simulink model "FINAL_MODEL"  (R2018a)
settings: Solver=FixedStepAuto  StartTime=startTime  StopTime=stopTime  FixedStep=stepSize  RelTol=1e-3
values from neighbouring files (symbols this model uses):
  burnCount = 2    [AA279D_FINAL.m]
  D2R = pi/180    (= 0.0174532925199)    [AA279D_FINAL.m]    (also in AA279D_PSET2.m; AA279D_PSET2_a_change.m; AA279D_PSET3.m; AA279D_PSET4.m)
  dV = zeros(3)    [AA279D_FINAL.m]    (also in AA279D_PSET2.m = [0;0;0]; AA279D_PSET2_a_change.m = [DVx;DVy;DVz]/stepSize; AA279D_PSET4.m = [0;0;0]; AA279D_hw4_v2.m = [0;0;0])
  dV_Timer = 5    [AA279D_FINAL.m]
  J2 = 1.081874*10^-3    (= 0.001081874)    [AA279D_FINAL.m]    (also in AA279D_PSET1.m; AA279D_PSET2.m; AA279D_PSET2_a_change.m; AA279D_PSET3.m)
  mu = 398600    [AA279D_FINAL.m]    (also in AA279D_PSET1.m; AA279D_PSET2.m; AA279D_PSET2_a_change.m; AA279D_PSET3.m)
  n = n_D    [AA279D_hw4.m]    (also in AA279D_hw4_v2.m = sqrt(mu/a^3); AA279D_hw5_dv.m = sqrt(mu/at^3); OE2ECI.m = sqrt(mu/a^3); TLE_Reader.m = revs_per_day*2*pi/(24*3600))
  Q_LQR = 1/(10)^2*eye(6)    [AA279D_FINAL.m]
  R_LQR = 1/(0.1)^2*eye(3)    [AA279D_FINAL.m]
  Re = 6378137*10^-3    (= 6378.137)    [AA279D_FINAL.m]    (also in AA279D_PSET1.m; AA279D_PSET2.m; AA279D_PSET2_a_change.m; AA279D_PSET3.m)
  roe = roe_out(end,:)    [AA279D_FINAL.m]    (also in AA279D_hw5.m = [0,100,50,100,30,200]/a*10e-4; AA279D_hw5_dv.m = [0,100,50,100,0,200]/a*10e-4; oe2roe.m = [da; deg2rad(dl); deg2rad(dex); deg2rad(dey); deg2rad(dix); )
  sig0 = sig_out(:,:,end)    [AA279D_FINAL.m]
  startTime = stopTime+stepSize    (= 12505)    [AA279D_FINAL.m]
  stepSize = 5    [AA279D_FINAL.m]    (also in AA279D_PSET1.m = 1; AA279D_PSET2.m; AA279D_PSET2_a_change.m = 1; AA279D_PSET3.m)
  uM = mod(uM,2*pi)    [AA279D_FINAL.m]
undefined symbols (not defined in the file or in its folder): r_eci_C, r_eci_D, v_eci_C, v_eci_D
libraries: simulink x3
settings Model: PacingRate=40  Creator=Christopher Covert  LastModifiedBy=Christopher Covert
settings SolverCC: AlgebraicLoopSolver=LineSearch

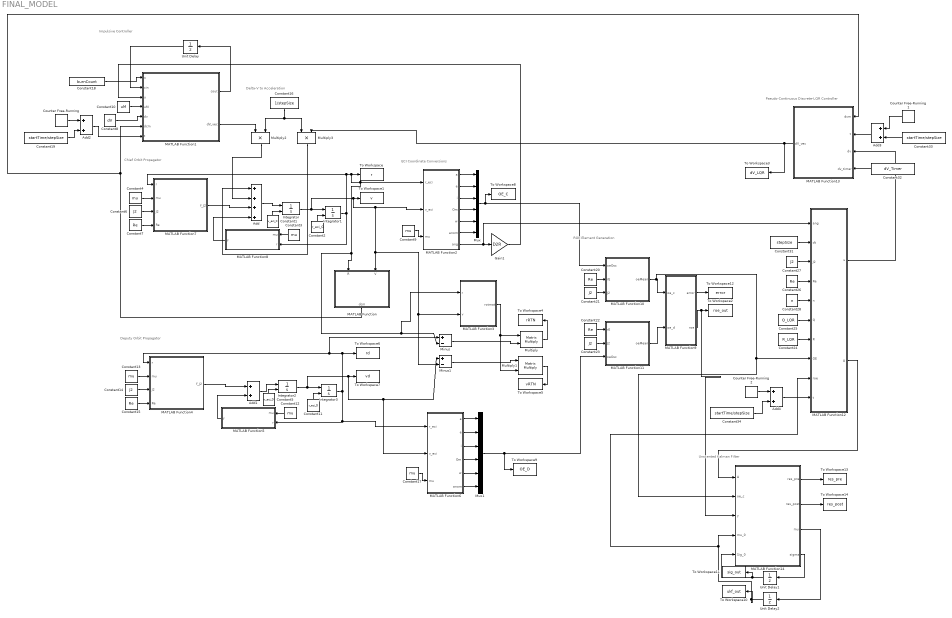
== system FINAL_MODEL ==
  note: Delta-V to Acceleration
  note: Unscented Kalman Filter
  note: Impulsive Controller
  note: Pseudo-Continuous Discrete-LQR Controller
  note: ROE Element Generation
  note: ECI Coordinate Conversions
  note: Chief Orbit Propagator
  note: Deputy Orbit Propagator
  Add : Sum  Inputs=++++
  Add{1..4} (4 alike) : Sum
  Constant1 : Constant  Value=v_eci_C
  Constant10 : Constant  Value=uM
  Constant11 : Constant  Value=r_eci_D
  Constant{3..4,9,12..13,17} (6 alike) : Constant  Value=mu
  Constant{6,14,21,23,27} (5 alike) : Constant  Value=J2
  Constant{7,15,20,22,26} (5 alike) : Constant  Value=Re
  Constant16 : Constant  Value=1/stepSize
  Constant18 : Constant  Value=burnCount
  Constant19 : Constant  Value=startTime/stepSize
  Constant2 : Constant  Value=r_eci_C
  Constant24 : Constant  Value=R_LQR
  Constant25 : Constant  Value=Q_LQR
  Constant28 : Constant  Value=n
  Constant31 : Constant  Value=stepSize
  Constant32 : Constant  Value=dV_Timer
  Constant33 : Constant  Value=startTime/stepSize
  Constant34 : Constant  Value=startTime/stepSize
  Constant5 : Constant  Value=v_eci_D
  Constant8 : Constant  Value=dV
  Counter Free-Running : simulink/Sources/Counter Free-Running  NumBits=16  tsamp=stepSize
  Counter Free-Running1 : simulink/Sources/Counter Free-Running  NumBits=16  tsamp=stepSize
  Counter Free-Running2 : simulink/Sources/Counter Free-Running  NumBits=16  tsamp=stepSize
  Gain1 : Gain  Gain=D2R
  Integrator{,1..3} (4 alike) : Integrator  InitialConditionSource=external
  MATLAB Function : MATLAB Function  TreatAsAtomicUnit=on
  MATLAB Function1 : MATLAB Function  TreatAsAtomicUnit=on
  MATLAB Function10 : MATLAB Function  TreatAsAtomicUnit=on
  MATLAB Function11 : MATLAB Function  TreatAsAtomicUnit=on
  MATLAB Function12 : MATLAB Function  TreatAsAtomicUnit=on
  MATLAB Function13 : MATLAB Function  TreatAsAtomicUnit=on
  MATLAB Function14 : MATLAB Function  TreatAsAtomicUnit=on
  MATLAB Function2 : MATLAB Function  TreatAsAtomicUnit=on
  MATLAB Function3 : MATLAB Function  TreatAsAtomicUnit=on
  MATLAB Function4 : MATLAB Function  TreatAsAtomicUnit=on
  MATLAB Function5 : MATLAB Function  TreatAsAtomicUnit=on
  MATLAB Function6 : MATLAB Function  TreatAsAtomicUnit=on
  MATLAB Function7 : MATLAB Function  TreatAsAtomicUnit=on
  MATLAB Function8 : MATLAB Function  TreatAsAtomicUnit=on
  MATLAB Function9 : MATLAB Function  TreatAsAtomicUnit=on
  Minus : Sum  Inputs=+-
  Minus1 : Sum  Inputs=+-
  Multiply : Product  Multiplication=Matrix(*)
  Multiply1 : Product  Multiplication=Matrix(*)
  Multiply2 : Product
  Multiply3 : Product
  Mux : Mux  Inputs=6
  Mux1 : Mux  Inputs=6
  To Workspace : ToWorkspace  VariableName=r  SampleTime=-1
      settings: Save2DSignal=2-D array (concatenate along first dimension)
  To Workspace1 : ToWorkspace  VariableName=v  SampleTime=-1
      settings: Save2DSignal=2-D array (concatenate along first dimension)
  To Workspace10 : ToWorkspace  VariableName=ukf_out  SampleTime=-1
      settings: Save2DSignal=2-D array (concatenate along first dimension)
  To Workspace11 : ToWorkspace  VariableName=sig_out  SampleTime=-1
  To Workspace12 : ToWorkspace  VariableName=error  SampleTime=-1
      settings: Save2DSignal=2-D array (concatenate along first dimension)
  To Workspace13 : ToWorkspace  VariableName=res_pre  SampleTime=-1
      settings: Save2DSignal=2-D array (concatenate along first dimension)
  To Workspace14 : ToWorkspace  VariableName=res_post  SampleTime=-1
      settings: Save2DSignal=2-D array (concatenate along first dimension)
  To Workspace2 : ToWorkspace  VariableName=roe_out  SampleTime=-1
      settings: Save2DSignal=2-D array (concatenate along first dimension)
  To Workspace3 : ToWorkspace  VariableName=dV_LQR  SampleTime=-1
      settings: Save2DSignal=2-D array (concatenate along first dimension)
  To Workspace4 : ToWorkspace  VariableName=rRTN  SampleTime=-1
      settings: Save2DSignal=2-D array (concatenate along first dimension)
  To Workspace5 : ToWorkspace  VariableName=vRTN  SampleTime=-1
      settings: Save2DSignal=2-D array (concatenate along first dimension)
  To Workspace6 : ToWorkspace  VariableName=rd  SampleTime=-1
      settings: Save2DSignal=2-D array (concatenate along first dimension)
  To Workspace7 : ToWorkspace  VariableName=vd  SampleTime=-1
      settings: Save2DSignal=2-D array (concatenate along first dimension)
  To Workspace8 : ToWorkspace  VariableName=OE_C  SampleTime=-1
      settings: Save2DSignal=2-D array (concatenate along first dimension)
  To Workspace9 : ToWorkspace  VariableName=OE_D  SampleTime=-1
      settings: Save2DSignal=2-D array (concatenate along first dimension)
  Unit Delay : UnitDelay  InputProcessing=Columns as channels (frame based)  SampleTime=-1
  Unit Delay1 : UnitDelay  InitialCondition=sig0  SampleTime=stepSize
  Unit Delay2 : UnitDelay  InitialCondition=roe  SampleTime=stepSize
  wires:
  Integrator/1 -> Integrator1/1, Minus1/2, MATLAB Function3/2(v), MATLAB Function/2(V), MATLAB Function2/2(v_eci), To Workspace1/1
  Constant3/1 -> MATLAB Function8/1(mu)
  Constant4/1 -> MATLAB Function7/2(mu)
  Constant6/1 -> MATLAB Function7/3(J2)
  Add/1 -> Integrator/1
  Constant7/1 -> MATLAB Function7/4(Re)
  MATLAB Function8/1(f) -> Add/4
  MATLAB Function7/1(f_J2) -> Add/3
  Constant1/1 -> Integrator/2
  Constant2/1 -> Integrator1/2
  Multiply2/1 -> Add/2
  MATLAB Function2/7(ang) -> MATLAB Function12/1(ang), Gain1/1
  Constant8/1 -> MATLAB Function1/5(dv)
  MATLAB Function1/2(dV_vec) -> Multiply2/1
  Constant9/1 -> MATLAB Function2/3(mu)
  Unit Delay/1 -> MATLAB Function1/2(cin)
  MATLAB Function1/1(cout) -> Unit Delay/1
  Constant10/1 -> MATLAB Function1/4(uM)
  MATLAB Function/1(dcm) -> MATLAB Function13/1(dcm), MATLAB Function1/6(dcm)
  MATLAB Function2/1(a) -> Mux/1
  MATLAB Function2/2(e) -> Mux/2
  MATLAB Function2/3(i) -> Mux/3
  MATLAB Function2/4(Om) -> Mux/4
  MATLAB Function2/5(w) -> Mux/5
  MATLAB Function2/6(anom) -> Mux/6
  Mux/1 -> To Workspace8/1, MATLAB Function10/1(oeOsc)
  Gain1/1 -> MATLAB Function1/3(u)
  Multiply1/1 -> To Workspace5/1
  Constant13/1 -> MATLAB Function4/2(mu)
  Constant15/1 -> MATLAB Function4/4(Re)
  Constant12/1 -> MATLAB Function5/1(mu)
  Constant5/1 -> Integrator2/2
  Constant11/1 -> Integrator3/2
  Constant14/1 -> MATLAB Function4/3(J2)
  Add1/1 -> Integrator2/1
  MATLAB Function4/1(f_J2) -> Add1/1
  MATLAB Function5/1(f) -> Add1/2
  Minus/1 -> Multiply/2
  Minus1/1 -> Multiply1/1
  Integrator1/1 -> MATLAB Function8/2(r), MATLAB Function7/1(r), MATLAB Function3/1(r), Minus/2, MATLAB Function/1(R), MATLAB Function2/1(r_eci), To Workspace/1
  MATLAB Function3/1(rotmat) -> Multiply1/2, Multiply/1
  Multiply/1 -> To Workspace4/1
  Constant16/1 -> Multiply2/2, Multiply3/1
  MATLAB Function6/6(anom) -> Mux1/6
  Integrator2/1 -> Integrator3/1, MATLAB Function6/2(v_eci), Minus1/1, To Workspace7/1
  Integrator3/1 -> MATLAB Function6/1(r_eci), MATLAB Function5/2(r), Minus/1, MATLAB Function4/1(r), To Workspace6/1
  Constant17/1 -> MATLAB Function6/3(mu)
  MATLAB Function6/3(i) -> Mux1/3
  MATLAB Function6/5(w) -> Mux1/5
  MATLAB Function6/1(a) -> Mux1/1
  MATLAB Function6/2(e) -> Mux1/2
  MATLAB Function6/4(Om) -> Mux1/4
  Counter Free-Running/1 -> Add2/1
  Constant19/1 -> Add2/2
  Add2/1 -> MATLAB Function1/7(t)
  Constant18/1 -> MATLAB Function1/1(n)
  MATLAB Function10/1(oeMean) -> MATLAB Function14/2(oe_c), MATLAB Function12/8(OE), MATLAB Function9/1(oe_c)
  Constant20/1 -> MATLAB Function10/2(rE)
  Constant21/1 -> MATLAB Function10/3(J2)
  Constant22/1 -> MATLAB Function11/1(rE)
  Constant23/1 -> MATLAB Function11/2(J2)
  Mux1/1 -> MATLAB Function11/3(oeOsc), To Workspace9/1
  MATLAB Function11/1(oeMean) -> MATLAB Function9/2(oe_d)
  MATLAB Function9/2(roe) -> MATLAB Function14/3(y), To Workspace2/1
  Constant24/1 -> MATLAB Function12/7(R)
  Constant25/1 -> MATLAB Function12/6(Q)
  Constant26/1 -> MATLAB Function12/4(Re)
  Constant27/1 -> MATLAB Function12/3(J2)
  MATLAB Function12/1(u) -> MATLAB Function13/3(dv)
  Constant28/1 -> MATLAB Function12/5(n)
  MATLAB Function13/1(dV_vec) -> To Workspace3/1, Multiply3/2
  Multiply3/1 -> Add/1
  Constant31/1 -> MATLAB Function12/2(dt)
  Constant33/1 -> Add3/2
  Counter Free-Running1/1 -> Add3/1
  Constant32/1 -> MATLAB Function13/4(dv_timer)
  Add3/1 -> MATLAB Function13/2(t)
  Constant34/1 -> Add4/2
  Counter Free-Running2/1 -> Add4/1
  Add4/1 -> MATLAB Function12/10(t)
  MATLAB Function14/4(sigma) -> Unit Delay1/1
  MATLAB Function14/3(mu) -> Unit Delay2/1
  Unit Delay1/1 -> MATLAB Function14/5(Sig_0), To Workspace11/1
  MATLAB Function12/2(A) -> MATLAB Function14/1(A)
  MATLAB Function14/1(res_pre) -> To Workspace13/1
  MATLAB Function14/2(res_post) -> To Workspace14/1
  Unit Delay2/1 -> To Workspace10/1, MATLAB Function12/9(roe), MATLAB Function14/4(mu_0)
  MATLAB Function9/1(error) -> To Workspace12/1

== matlab function FINAL_MODEL/MATLAB Function1 ==
  data: n input; cin input; u input; uM input; cout output; dv input; dV_vec output; dcm input; t input
function [cout,dV_vec] = impulse_man(n,cin,u,uM,dv,dcm,t)

i = cin+1;

if double(t) == 116 && n == 1
    dV_vec = dcm*[dv(1,1);dv(2,1);dv(3,1)];
%     fprintf('Completed Burn No.%0.0f at t = %0.2f\n',i,double(t));
    cout = cin+1;
elseif n == 2 && double(t) == 3519
    dV_vec = dcm*[dv(1,1);dv(2,1);dv(3,1)];
%     fprintf('Completed Burn No.%0.0f at t = %0.2f\n',i,double(t));
    cout = cin+1;
elseif double(t) == 830 && n == 1
    dV_vec = -dcm*[dv(1,2);dv(2,2);dv(3,2)];
%     fprintf('Completed Burn No.%0.0f at t = %0.2f\n',i,double(t));
    cout = cin+1;
elseif  n == 2 && double(t) == 4130
    dV_vec = -dcm*[dv(1,2);dv(2,2);dv(3,2)]*1.1;
%     fprintf('Completed Burn No.%0.0f at t = %0.2f\n',i,double(t));
    cout = cin+1;
elseif double(t) == 1385 && n == 1
    dV_vec = -dcm*[dv(1,3);dv(2,3);dv(3,3)];
%     fprintf('Completed Burn No.%0.0f at t = %0.2f\n',i,double(t));
    cout = cin+1;
elseif  n == 2 && double(t) == 4673
    dV_vec = -dcm*[dv(1,3);dv(2,3);dv(3,3)]*0.93;
%     fprintf('Completed Burn No.%0.0f at t = %0.2f\n',i,double(t));
    cout = cin+1;
else
    dV_vec = [0;0;0];
    cout = cin;
end

end

== matlab function FINAL_MODEL/MATLAB Function2 ==
  data: a output; e output; i output; Om output; r_eci input; v_eci input; mu input; w output; anom output; ang output
function [a, e, i, Om, w, anom, ang] = ECI2OE(r_eci, v_eci, mu)
% ECI2OE Converts r and v in the ECI frame to orbital elements
%
% Inputs:
%   r_eci - 3x1 vector of radius in ECI frame [km]
%   v_eci - 3x1 vector of velocity in ECI frame [km]
%   mu    - gravitational parameter of central body [km^3/s^2]
%
% Outputs:
%   p     - semi-lactus rectum of orbit [km]
%   a     - semi-major axis of orbit [km]
%   e     - eccentricity of orbit
%   i     - inclination of orbit [deg]
%   Om    - right ascension of the ascending node [deg]
%   w     - argument of periapsis [deg]
%   v     - true anomaly [deg]
%   ang   - extra placeholder angle for special cases [deg]
%
% This function is able to handle any orbit type, including equatorial and
% circular orbits. The output ang will output the following values for each
% orbit type
%   1) Elliptical equatorial
%       Longitude of periapsis, Pi = Om + w
%   2) Circular inclined
%       Argument of latitude, u = w + anom
%   3) Circular equatorial
%       True latitude, lambda = Om + w + anom
% Otherwise, ang will be undefined (NaN)

r = norm(r_eci);
v = norm(v_eci);

% Create all necessary vectors
hVec = cross(r_eci, v_eci);
h = norm(hVec);

nVec = cross([0, 0, 1], hVec);
n = norm(nVec);

eVec = (1/mu)*((v^2 - mu/r)*r_eci - dot(r_eci, v_eci)*v_eci);
e = norm(eVec);

% Compute the size of the orbit
mechEnergy = 0.5*v^2 - mu/r;

if e ~= 1
    a = -mu/(2*mechEnergy);
else
    a = inf; % Semi-major axis undefined for parabolas
end

% Compute the orientation of the orbit
i = rad2deg(acos(hVec(3)/h));
Om = rad2deg(acos(nVec(1)/n));
w = rad2deg(acos(dot(nVec, eVec)/(n*e)));
anom = rad2deg(acos(dot(eVec, r_eci)/(e*r)));

% Place angles in the correct domains
if nVec(2) < 0
    Om = 360 - Om;
end
if eVec(3) < 0
    w = 360 - w;
end
if dot(r_eci, v_eci) < 0
    anom = 360 - anom;
end

% Account for any special cases
if i == 0 && e ~= 0 % Elliptical equatorial
    % Provide the longitude of periapsis (PI = Om + w)
    ang = rad2deg(acos(eVec(1)/e));

    if eVec(2) < 0
        ang = 360 - ang;
    end
elseif i ~= 0 && e == 0 % Circular inclined
    % Provide the argument of latitude (u = w + anom)
    ang = rad2deg(acos(dot(nVec, r_eci)/(n*r)));

    if r_eci(3) < 0
        ang = 360 - ang;
    end
elseif i == 0 && e == 0 % Circular equatorial
    % Provide the true latitude (lambda = Om + w + anom)
    ang = rad2deg(acos(r_eci(1)/r));

    if r_eci(2) < 0
        ang = 360 - ang;
    end
else
    % Default output for ang
    ang = NaN;
end

ang = mod(w + anom,360);


end

== matlab function FINAL_MODEL/MATLAB Function ==
  data: R input; dcm output; V input
function dcm = RTN2ECI(R, V)
% RTN2ECI Computes rotation matrices from RTN frame to inertial frame
%
% Inputs:
%   R - 3xn inertial position vectors
%   V - 3xn inertial velocity vectors
%
% Outputs:
%   dcm - 3x3xn rotation matrices from inertial to RTN

% Set up the input matrices as a (3 x n) series of column vectors
if size(R, 2) == 3 && size(R, 1) ~= 3
    R = R.';
end

if size(V, 2) == 3 && size(V, 1) ~= 3
    V = V.';
end

% Check input sizes
numPos = size(R, 2);
numVel = size(V, 2);

if size(R, 1) ~= 3
    error('Position vectors must come in the form of 3xn column vectors');
elseif size(V, 1) ~= 3
    error('Velocity vectors must come in the form of 3xn column vectors');
elseif numPos ~= numVel
    error('Must provide the same number of position and velocity vectors');
end

dcm = zeros(3, 3, numPos);

for i = 1:numPos
    rVec = R(:, i)./norm(R(:, i));
    
    H = cross(R(:, i), V(:, i));
    nVec = H./norm(H);
    
    T = cross(nVec, rVec);
    tVec = T./norm(T);
    
    dcm(:, :, i) = [rVec, tVec, nVec];
end

end

== matlab function FINAL_MODEL/MATLAB Function7 ==
  data: r input; f_J2 output; mu input; J2 input; Re input
function f_J2 = J2_Accel(r,mu,J2,Re)

f_J2 = mu*r/(norm(r)^3).*...
    [3/2*J2*(Re/norm(r))^2*(5*(r(3)^2)/(norm(r)^2)-1);...
    3/2*J2*(Re/norm(r))^2*(5*(r(3)^2)/(norm(r)^2)-1);...
    3/2*J2*(Re/norm(r))^2*(5*(r(3)^2)/(norm(r)^2)-3)];

== matlab function FINAL_MODEL/MATLAB Function8 ==
  data: mu input; f output; r input
function f = FODE_NUM_PROP(mu,r)

f = -mu*r/(norm(r)^3);

== matlab function FINAL_MODEL/MATLAB Function3 ==
  data: r input; rotmat output; v input
function rotmat = ECI2RTN( r,v)

r=reshape(r,1,3);
v=reshape(v,1,3);
unitr=r/norm(r);
unitn=cross(r,v)/norm(cross(r,v));
unitt=cross(unitn,r)/norm(cross(unitn,r));
rotmat=[unitr;
    unitt;
    unitn];

end

== matlab function FINAL_MODEL/MATLAB Function4 ==
  data: r input; f_J2 output; mu input; J2 input; Re input
function f_J2 = J2_Accel(r,mu,J2,Re)

f_J2 = mu*r/(norm(r)^3).*...
    [3/2*J2*(Re/norm(r))^2*(5*(r(3)^2)/(norm(r)^2)-1);...
    3/2*J2*(Re/norm(r))^2*(5*(r(3)^2)/(norm(r)^2)-1);...
    3/2*J2*(Re/norm(r))^2*(5*(r(3)^2)/(norm(r)^2)-3)];

== matlab function FINAL_MODEL/MATLAB Function5 ==
  data: mu input; f output; r input
function f = FODE_NUM_PROP(mu,r)

f = -mu*r/(norm(r)^3);

== matlab function FINAL_MODEL/MATLAB Function6 ==
  data: a output; e output; i output; Om output; r_eci input; v_eci input; mu input; w output; anom output
function [a, e, i, Om, w, anom] = ECI2OE(r_eci, v_eci, mu)
% ECI2OE Converts r and v in the ECI frame to orbital elements
%
% Inputs:
%   r_eci - 3x1 vector of radius in ECI frame [km]
%   v_eci - 3x1 vector of velocity in ECI frame [km]
%   mu    - gravitational parameter of central body [km^3/s^2]
%
% Outputs:
%   p     - semi-lactus rectum of orbit [km]
%   a     - semi-major axis of orbit [km]
%   e     - eccentricity of orbit
%   i     - inclination of orbit [deg]
%   Om    - right ascension of the ascending node [deg]
%   w     - argument of periapsis [deg]
%   v     - true anomaly [deg]
%   ang   - extra placeholder angle for special cases [deg]
%
% This function is able to handle any orbit type, including equatorial and
% circular orbits. The output ang will output the following values for each
% orbit type
%   1) Elliptical equatorial
%       Longitude of periapsis, Pi = Om + w
%   2) Circular inclined
%       Argument of latitude, u = w + anom
%   3) Circular equatorial
%       True latitude, lambda = Om + w + anom
% Otherwise, ang will be undefined (NaN)

r = norm(r_eci);
v = norm(v_eci);

% Create all necessary vectors
hVec = cross(r_eci, v_eci);
h = norm(hVec);

nVec = cross([0, 0, 1], hVec);
n = norm(nVec);

eVec = (1/mu)*((v^2 - mu/r)*r_eci - dot(r_eci, v_eci)*v_eci);
e = norm(eVec);

% Compute the size of the orbit
mechEnergy = 0.5*v^2 - mu/r;

if e ~= 1
    a = -mu/(2*mechEnergy);
else
    a = inf; % Semi-major axis undefined for parabolas
end

% Compute the orientation of the orbit
i = rad2deg(acos(hVec(3)/h));
Om = rad2deg(acos(nVec(1)/n));
w = rad2deg(acos(dot(nVec, eVec)/(n*e)));
anom = rad2deg(acos(dot(eVec, r_eci)/(e*r)));

% Place angles in the correct domains
if nVec(2) < 0
    Om = 360 - Om;
end
if eVec(3) < 0
    w = 360 - w;
end
if dot(r_eci, v_eci) < 0
    anom = 360 - anom;
end

% Account for any special cases
if i == 0 && e ~= 0 % Elliptical equatorial
    % Provide the longitude of periapsis (PI = Om + w)
    ang = rad2deg(acos(eVec(1)/e));

    if eVec(2) < 0
        ang = 360 - ang;
    end
elseif i ~= 0 && e == 0 % Circular inclined
    % Provide the argument of latitude (u = w + anom)
    ang = rad2deg(acos(dot(nVec, r_eci)/(n*r)));

    if r_eci(3) < 0
        ang = 360 - ang;
    end
elseif i == 0 && e == 0 % Circular equatorial
    % Provide the true latitude (lambda = Om + w + anom)
    ang = rad2deg(acos(r_eci(1)/r));

    if r_eci(2) < 0
        ang = 360 - ang;
    end
else
    % Default output for ang
    ang = NaN;
end

ang = mod(w + anom,360);


end

== matlab function FINAL_MODEL/MATLAB Function9 ==
  data: error output; oe_c input; roe output; oe_d input
function [error,roe]  = oe2roe(oe_c, oe_d)
% oe2roe Converts absolute to relative orbital elements
%
% Inputs:
%       oe_c - chief orbital elements (all angles in degrees)
%              [a, e, i, Om, w, anom]
%       oe_d - deputy orbital elements (all angles in degrees)
%              [ad, ed, id, Omd, wd, anomd]
%   anomFlag - (optional) flag indicating whether the provided anomalies
%              are true (1 - default) or mean (0). The output set of deputy
%              OEs will match.
%
% Outputs:
%        roe - quasi-non singular relative orbital elements

% Parse out the chief and deputy orbit elements
a = oe_c(1);
e = oe_c(2);
i = oe_c(3);
Om = oe_c(4);
w = oe_c(5);
anom = oe_c(6);

ad = oe_d(1);
ed = oe_d(2);
id = oe_d(3);
Omd = oe_d(4);
wd = oe_d(5);
anomd = oe_d(6);

M = rad2deg(E2M(anom2E(deg2rad(anom), e), e));
Md = rad2deg(E2M(anom2E(deg2rad(anomd), ed), ed));

u = w + M;
ud = wd + Md;

Om_diff = Omd-Om;

if Om_diff < -340
    Om_diff = Om_diff + 360;
end

% Compute D'Amico's quasi-nonsingular ROEs
da = (ad - a)./a;
dl = (ud - u) + (Om_diff).*cosd(i);
dex = ed.*cosd(wd) - e.*cosd(w);
dey = ed.*sind(wd) - e.*sind(w);
dix = id - i;
diy = (Om_diff).*sind(i);

error = Omd-Om;

if dl > 340
    dl = dl-360;
end

if dl < -340
    dl = dl+360;
end

roe = [da; deg2rad(dl); deg2rad(dex); deg2rad(dey); deg2rad(dix); deg2rad(diy)];

end

== matlab function FINAL_MODEL/MATLAB Function10 ==
  data: oeOsc input; oeMean output; rE input; J2 input
function oeMean = osc2mean(oeOsc, rE, J2)
% osc2mean Converts osculating orbit elements to mean orbit elements
%
%   This method is based on the first-order mapping provided in Schaub
%   Appendix G. Note that it only accounts for first-order J2 terms, and
%   thus cannot be applied to any general set of osculating orbit elements.
%
%   Note that this method fails for perfectly circular/equatorial orbits.
%   It is recommended that a very small offset (e.g. 1E-6) is introduced to
%   the eccentricity/inclination if one wishes to evaluate the conversion
%   for a circular/equatorial orbit.
%
% Inputs:
%   oeOsc - 6x1 vector of osculating orbit elements:
%          a - semi-major axis of osculating orbit [km]
%          e - eccentricity of osculating orbit
%          i - inclination of osculating orbit [deg]
%         Om - osculating right ascension of the ascending node [deg]
%          w - osculating argument of periapsis [deg]
%       anom - osculating true anomaly [deg]
%     rE - equatorial radius of central body [km]
%     J2 - central body J2 term
%
% Outputs:
%   oeMean - 6x1 vector of mean orbit elements:
%          a - semi-major axis of mean orbit [km]
%          e - eccentricity of mean orbit
%          i - inclination of mean orbit [deg]
%         Om - mean right ascension of the ascending node [deg]
%          w - mean argument of periapsis [deg]
%       anom - mean true anomaly [deg]

% Parse out the osculating orbit elements
a = oeOsc(1);
e = oeOsc(2);
i = oeOsc(3);
Om = oeOsc(4);
w = oeOsc(5);
anom = oeOsc(6);

% Convert all input elements from degrees to radian
i = deg2rad(i);
Om = deg2rad(Om);
w = deg2rad(w);
anom = deg2rad(anom);

% Wrap angles between -pi and pi (robustness)
i = mod(i, pi);
Om = mod(Om, 2*pi) - (Om > pi)*2*pi;
w = mod(w, 2*pi) - (w > pi)*2*pi;
%anom = mod(anom, 2*pi) - (anom > pi)*2*pi;

% Convert the true anomaly to mean anomaly
E = anom2E(anom, e);
M = E2M(E, e);

% Gather necessary constants
g2 = -(J2/2)*(rE/a)^2; % Note: minus sign indicates osc -> mean
eta = sqrt(1 - e^2);
g2_p = g2/eta^4;

a_r = (1 + e*cos(anom))/eta^2;

% Equation G.304:
de1 = (g2_p/8)*e*eta^2*(1 - 11*cos(i)^2 - ...
    40*(cos(i)^4/(1 - 5*cos(i)^2)))*cos(2*w);
de2 = g2*((3*cos(i)^2 - 1)/eta^6)*(e*eta + e/(1 + eta) + ...
    3*cos(anom) + 3*e*cos(anom)^2 + e^2*cos(anom)^3);
de3 = g2*(3*(1 - cos(i)^2)/eta^6)*(e + 3*cos(anom) + ...
    3*e*cos(anom)^2 + e^2*cos(anom)^3)*cos(2*w + 2*anom);
de4 = -g2_p*(1 - cos(i)^2)*(3*cos(2*w + anom) + cos(2*w + 3*anom));

de = de1 + (eta^2)/2*(de2 + de3 + de4);

% Equation G.305:
di1 = -(e*de1)/(eta^2*tan(i));
di2 = g2_p/2*cos(i)*sqrt(1 - cos(i)^2)*(3*cos(2*w + 2*anom) + ...
    3*e*cos(2*w + anom) + e*cos(2*w + 3*anom));

di = di1 + di2;

% Equation G.306:
dL0 = M + w + Om;
dL1 = (g2_p/8)*eta^3*(1 - 11*cos(i)^2 - ...
    40*(cos(i)^4/(1 - 5*cos(i)^2)));
dL2 = -(g2_p/16)*(2 + e^2 - 11*(2 + 3*e^2)*cos(i)^2 - ...
    40*(2 + 5*e^2)*(cos(i)^4/(1 - 5*cos(i)^2)) - ...
    400*e^2*(cos(i)^6/(1 - 5*cos(i)^2)^2));
dL3 = (g2_p/4)*(-6*(1 - 5*cos(i)^2)*(anom - M + e*sin(anom)) + ...
    (3 - 5*cos(i)^2)*(3*sin(2*w + 2*anom) + 3*e*sin(2*w + anom) + ...
    e*sin(2*w + 3*anom)));
dL4 = -(g2_p/8)*e^2*cos(i)*(11 + 80*(cos(i)^2/(1 - 5*cos(i)^2)) +...
    200*(cos(i)^4/(1 - 5*cos(i)^2)^2));
dL5 = -(g2_p/2)*cos(i)*(6*(anom - M + e*sin(anom)) - ...
    3*sin(2*w + 2*anom) - 3*e*sin(2*w + anom) - e*sin(2*w + 3*anom));

dL = dL0 + dL1 + dL2 + dL3 + dL4 + dL5;

% Equation G.307:
edM1 = (g2_p/8)*e*eta^3*(1 - 11*cos(i)^2 - ...
    40*(cos(i)^4/(1 - 5*cos(i)^2)));
edM2 = 2*(3*cos(i)^2 - 1)*((a_r*eta)^2 + a_r + 1)*sin(anom);
edM3 = 3*(1 - cos(i)^2)*((-(a_r*eta)^2 - a_r + 1)*sin(2*w + anom) + ...
    ((a_r*eta)^2 + a_r + 1/3)*sin(2*w + 3*anom));

edM = edM1 - (g2_p/4)*eta^3*(edM2 + edM3);

% Equation G.308
dOm1 = -(g2_p/8)*e^2*cos(i)*(11 + 80*(cos(i)^2/(1 - 5*cos(i)^2)) +...
    200*(cos(i)^4/(1 - 5*cos(i)^2)^2));
dOm2 = -(g2_p/2)*cos(i)*(6*(anom - M + e*sin(anom)) - ...
    3*sin(2*w + 2*anom) - 3*e*sin(2*w + anom) - e*sin(2*w + 3*anom));

dOm = dOm1 + dOm2;

% Equations G.309-310, G.313-314
d1 = (e + de)*sin(M) + edM*cos(M);
d2 = (e + de)*cos(M) - edM*sin(M);
d3 = (sin(i/2) + cos(i/2)*(di/2))*sin(Om) + sin(i/2)*dOm*cos(Om);
d4 = (sin(i/2) + cos(i/2)*(di/2))*cos(Om) - sin(i/2)*dOm*sin(Om);

% Compute all of the mean orbit elements using the previously computed
% parameters
aM = a + a*g2*((3*cos(i)^2 - 1)*(a_r^3 - 1/eta^3) + ...
    3*(1 - cos(i)^2)*a_r^3*cos(2*w + 2*anom));
eM = sqrt(d1^2 + d2^2);
iM = 2*asin(sqrt(d3^2 + d4^2));
OmM = mod(atan2(d3, d4), 2*pi);
MM = mod(atan2(d1, d2), 2*pi);
wM = mod(dL - MM - OmM, 2*pi);

% Convert the mean mean anomaly to mean true anomaly
EM = M2E(MM, e, 1E-9);
anomM = E2anom(EM, e);

% Convert all mean orbit elements from radians to degrees
iM = rad2deg(iM);
OmM = rad2deg(OmM);
wM = rad2deg(wM);
anomM = rad2deg(anomM);

% Gather the mean orbit elements into one vector
oeMean = [aM; eM; iM; OmM; wM; anomM];

end

== matlab function FINAL_MODEL/MATLAB Function11 ==
  data: rE input; J2 input; oeOsc input; oeMean output
function oeMean = osc2mean(  rE, J2, oeOsc)
% osc2mean Converts osculating orbit elements to mean orbit elements
%
%   This method is based on the first-order mapping provided in Schaub
%   Appendix G. Note that it only accounts for first-order J2 terms, and
%   thus cannot be applied to any general set of osculating orbit elements.
%
%   Note that this method fails for perfectly circular/equatorial orbits.
%   It is recommended that a very small offset (e.g. 1E-6) is introduced to
%   the eccentricity/inclination if one wishes to evaluate the conversion
%   for a circular/equatorial orbit.
%
% Inputs:
%   oeOsc - 6x1 vector of osculating orbit elements:
%          a - semi-major axis of osculating orbit [km]
%          e - eccentricity of osculating orbit
%          i - inclination of osculating orbit [deg]
%         Om - osculating right ascension of the ascending node [deg]
%          w - osculating argument of periapsis [deg]
%       anom - osculating true anomaly [deg]
%     rE - equatorial radius of central body [km]
%     J2 - central body J2 term
%
% Outputs:
%   oeMean - 6x1 vector of mean orbit elements:
%          a - semi-major axis of mean orbit [km]
%          e - eccentricity of mean orbit
%          i - inclination of mean orbit [deg]
%         Om - mean right ascension of the ascending node [deg]
%          w - mean argument of periapsis [deg]
%       anom - mean true anomaly [deg]

% Parse out the osculating orbit elements
a = oeOsc(1);
e = oeOsc(2);
i = oeOsc(3);
Om = oeOsc(4);
w = oeOsc(5);
anom = oeOsc(6);

% Convert all input elements from degrees to radian
i = deg2rad(i);
Om = deg2rad(Om);
w = deg2rad(w);
anom = deg2rad(anom);

% Wrap angles between -pi and pi (robustness)
i = mod(i, pi);
Om = mod(Om, 2*pi) - (Om > pi)*2*pi;
w = mod(w, 2*pi) - (w > pi)*2*pi;
%anom = mod(anom, 2*pi) - (anom > pi)*2*pi;

% Convert the true anomaly to mean anomaly
E = anom2E(anom, e);
M = E2M(E, e);

% Gather necessary constants
g2 = -(J2/2)*(rE/a)^2; % Note: minus sign indicates osc -> mean
eta = sqrt(1 - e^2);
g2_p = g2/eta^4;

a_r = (1 + e*cos(anom))/eta^2;

% Equation G.304:
de1 = (g2_p/8)*e*eta^2*(1 - 11*cos(i)^2 - ...
    40*(cos(i)^4/(1 - 5*cos(i)^2)))*cos(2*w);
de2 = g2*((3*cos(i)^2 - 1)/eta^6)*(e*eta + e/(1 + eta) + ...
    3*cos(anom) + 3*e*cos(anom)^2 + e^2*cos(anom)^3);
de3 = g2*(3*(1 - cos(i)^2)/eta^6)*(e + 3*cos(anom) + ...
    3*e*cos(anom)^2 + e^2*cos(anom)^3)*cos(2*w + 2*anom);
de4 = -g2_p*(1 - cos(i)^2)*(3*cos(2*w + anom) + cos(2*w + 3*anom));

de = de1 + (eta^2)/2*(de2 + de3 + de4);

% Equation G.305:
di1 = -(e*de1)/(eta^2*tan(i));
di2 = g2_p/2*cos(i)*sqrt(1 - cos(i)^2)*(3*cos(2*w + 2*anom) + ...
    3*e*cos(2*w + anom) + e*cos(2*w + 3*anom));

di = di1 + di2;

% Equation G.306:
dL0 = M + w + Om;
dL1 = (g2_p/8)*eta^3*(1 - 11*cos(i)^2 - ...
    40*(cos(i)^4/(1 - 5*cos(i)^2)));
dL2 = -(g2_p/16)*(2 + e^2 - 11*(2 + 3*e^2)*cos(i)^2 - ...
    40*(2 + 5*e^2)*(cos(i)^4/(1 - 5*cos(i)^2)) - ...
    400*e^2*(cos(i)^6/(1 - 5*cos(i)^2)^2));
dL3 = (g2_p/4)*(-6*(1 - 5*cos(i)^2)*(anom - M + e*sin(anom)) + ...
    (3 - 5*cos(i)^2)*(3*sin(2*w + 2*anom) + 3*e*sin(2*w + anom) + ...
    e*sin(2*w + 3*anom)));
dL4 = -(g2_p/8)*e^2*cos(i)*(11 + 80*(cos(i)^2/(1 - 5*cos(i)^2)) +...
    200*(cos(i)^4/(1 - 5*cos(i)^2)^2));
dL5 = -(g2_p/2)*cos(i)*(6*(anom - M + e*sin(anom)) - ...
    3*sin(2*w + 2*anom) - 3*e*sin(2*w + anom) - e*sin(2*w + 3*anom));

dL = dL0 + dL1 + dL2 + dL3 + dL4 + dL5;

% Equation G.307:
edM1 = (g2_p/8)*e*eta^3*(1 - 11*cos(i)^2 - ...
    40*(cos(i)^4/(1 - 5*cos(i)^2)));
edM2 = 2*(3*cos(i)^2 - 1)*((a_r*eta)^2 + a_r + 1)*sin(anom);
edM3 = 3*(1 - cos(i)^2)*((-(a_r*eta)^2 - a_r + 1)*sin(2*w + anom) + ...
    ((a_r*eta)^2 + a_r + 1/3)*sin(2*w + 3*anom));

edM = edM1 - (g2_p/4)*eta^3*(edM2 + edM3);

% Equation G.308
dOm1 = -(g2_p/8)*e^2*cos(i)*(11 + 80*(cos(i)^2/(1 - 5*cos(i)^2)) +...
    200*(cos(i)^4/(1 - 5*cos(i)^2)^2));
dOm2 = -(g2_p/2)*cos(i)*(6*(anom - M + e*sin(anom)) - ...
    3*sin(2*w + 2*anom) - 3*e*sin(2*w + anom) - e*sin(2*w + 3*anom));

dOm = dOm1 + dOm2;

% Equations G.309-310, G.313-314
d1 = (e + de)*sin(M) + edM*cos(M);
d2 = (e + de)*cos(M) - edM*sin(M);
d3 = (sin(i/2) + cos(i/2)*(di/2))*sin(Om) + sin(i/2)*dOm*cos(Om);
d4 = (sin(i/2) + cos(i/2)*(di/2))*cos(Om) - sin(i/2)*dOm*sin(Om);

% Compute all of the mean orbit elements using the previously computed
% parameters
aM = a + a*g2*((3*cos(i)^2 - 1)*(a_r^3 - 1/eta^3) + ...
    3*(1 - cos(i)^2)*a_r^3*cos(2*w + 2*anom));
eM = sqrt(d1^2 + d2^2);
iM = 2*asin(sqrt(d3^2 + d4^2));
OmM = mod(atan2(d3, d4), 2*pi);
MM = mod(atan2(d1, d2), 2*pi);
wM = mod(dL - MM - OmM, 2*pi);

% Convert the mean mean anomaly to mean true anomaly
EM = M2E(MM, e, 1E-9);
anomM = E2anom(EM, e);

% Convert all mean orbit elements from radians to degrees
iM = rad2deg(iM);
OmM = rad2deg(OmM);
wM = rad2deg(wM);
anomM = rad2deg(anomM);

% Gather the mean orbit elements into one vector
oeMean = [aM; eM; iM; OmM; wM; anomM];

end

== matlab function FINAL_MODEL/MATLAB Function12 ==
  data: ang input; dt input; u output; J2 input; Re input; n input; Q input; R input; OE input; roe input; t input; A output
function [u,A]  = dlqr_iter(ang,dt,J2,Re,n,Q,R,OE,roe,t)

a = OE(1);
e = OE(2);
i = OE(3);
RAAN = OE(4);
w = OE(5);
anom = OE(6);
% ang = w+anom;

nu = (-3/2)*n;
eta = sqrt(1-e^2);
gamma = J2/2*(Re/a)^2*(1/eta^4);
psidot = (3/2)*n*gamma*(5*cosd(i)^2-1);
mu = -21/2*n*gamma*sind(2*i);
lam = 3*n*gamma*sind(i)^2;

A = [1,0,0,0,0,0;...
    nu*dt,1,0,0,mu*dt,0;...
    0,0,1,-psidot*dt,0,0;...
    0,0,psidot*dt,1,0,0;...
    0,0,0,0,1,0;...
    0,0,0,0,lam*dt,1];

B = 1/(a*n)*[0,2,0;...
    -2,0,0;...
    sind(ang),2*cosd(ang),0;...
    -cosd(ang),2*sind(ang),0;...
    0,0,cosd(ang);...
    0,0,sind(ang)];

coder.extrinsic('dlqr');
K = zeros(3,6);
[K,~,~] = dlqr(A,B,Q,R);

if double(t) > 1386 && double(t) < 3445
    OE_d = [a+350/1000,e,i+0.0001,RAAN+0.0001,w+0.0001,anom-0.0001];
    roe_des = oe2roe(OE, OE_d);
elseif double(t) > 4965
    OE_d = [a+10/1000,e,i,RAAN,w,anom];
    roe_des = oe2roe(OE, OE_d);
else
    roe_des = roe;
end

u = -K*(roe-roe_des);

== matlab function FINAL_MODEL/MATLAB Function13 ==
  data: dcm input; t input; dv input; dV_vec output; dv_timer input
function dV_vec  = impulse_man(dcm,t,dv,dv_timer)

if double(t) > 1400 && double(t) < 3500 && mod(double(t),dv_timer) == 0
    dV_vec = dcm*[dv(1);dv(2);dv(3)]/100;
elseif double(t) > 4098 && mod(double(t),dv_timer) == 0
    dV_vec = dcm*[dv(1);dv(2);dv(3)]*0;
else
    dV_vec = [0;0;0];
end

end

== matlab function FINAL_MODEL/MATLAB Function14 ==
  settings: updateMethod=DISCRETE  sampleTime=stepSize
  data: res_pre output; res_post output; A input; oe_c input; y input; mu_0 input; mu output; sigma output; Sig_0 input
function [res_pre,res_post,mu,sigma] = ukf(A, oe_c, y, mu_0, Sig_0)
nX = length(mu_0');
nY = length(y);
J2 = 0.00108263;

Q = 0.1*eye(6);
R = 0.1*eye(6);
lam = 2;

V = (rand(1,6)*0.0000001*eye(6))';
y = y + V;

% perform UT
[xSig, wt] = UT(lam, nX, mu_0, Sig_0);

%
% predict
%
xSigTemp = zeros(nX, 2*nX+1);
for i = 1:(2*nX+1)
    STM = A;
    xSigTemp(:,i) = STM * xSig(:,i);
end

% perform inv UT
muNew = xSigTemp*wt';
SigNew = zeros(nX,nX);
for i = 1:(2*nX+1)
    SigNew = SigNew + wt(i)*( xSigTemp(:,i) - muNew )*...
        (xSigTemp(:,i) - muNew)';
end
%%%
SigNew = SigNew + Q;
%%%

% perform UT on predicted dist
[xSigNew, wtNew] = UT(lam, nX, muNew, SigNew);

% use new sigma points to predict measurement
yhatSig = xSig;
yhat = yhatSig*wtNew';

%
% update
%
SigYY = zeros(nY,nY);
SigXY = zeros(nX,nY);
for i = 1:(2*nX+1)
    SigYY = SigYY + wt(i)*(yhatSig(:,i) - yhat)*(yhatSig(:,i) - yhat)';
    SigXY = SigXY + wt(i)*(xSigNew(:,i) - muNew)*(yhatSig(:,i) - yhat)';
end
SigYY = SigYY + R;

Kukf = SigXY / SigYY;
mu = muNew + Kukf*(y - yhat);
sigma = SigNew - Kukf*SigXY';

% calculate residuals
res_pre = y - yhat;
yhat_post = mu;
res_post = y - yhat_post;

%%%
% Unscented Transform
%%%
    function [xSig, wt] = UT(lam, n, mu, Sig)
        xSig = zeros(n,2*n+1);
        wt = zeros(1,2*n+1);
        xSig(:,1) = mu;
        wt(1) = lam / (n + lam);
%         coder.extrinsic('sqrtm');
%         sqrtSig = zeros(n, n);
%         sqrtSig = sqrtm(Sig);
        sqrtSig = chol(Sig);
        for j = 1:n
            xSig(:,j+1) = mu + sqrt(n+lam)*sqrtSig(:,j);
            xSig(:,n+1+j) = mu - sqrt(n+lam)*sqrtSig(:,j);
            wt(j+1) = 1 / (2*(n+lam));
            wt(n+1+j) = wt(j+1);
        end
    end
end
